simulink model "c6_formation"  (R2021b)
settings: Solver=FixedStepDiscrete  StartTime=0.0  StopTime=Inf  FixedStep=sampleTime  RelTol=1e-3  EnableMultiTasking=on
PreLoadFcn:
  | %load emptyMap
  | 
  | % Lidar parameters
  | sensorOffset = [0,0];
  | scanAngles = -pi:pi/6:pi;
  | maxRange = 0.25;
InitFcn:
  | sampleTime = 0.05;
  | nMedianSize=3;
  | 
  | % Robot parameters
  | wheelRadius = 0.0335;
  | robotRadius = 0.116/2;
  | 
  | %角速度坐标
  | ks=1;
  | 
  | % Lidar parameters
  | sensorOffset = [0,0];
  | scanAngles = -pi/3:pi/36:pi/3;
  | maxRange = 0.2;
  | 
  | %车初始位置
  | init_pose_1=[1  1.3  pi/2]';
  | init_pose_2=[0.85 1  pi/2]';
  | init_pose_3=[1.15 1  pi/2]';
  | init_pose_4=[0.7  0.7 pi/2]';
  | init_pose_5=[1  0.7 pi/2]';
  | init_pose_6=[1.3 0.7  pi/2]';
  | 
  | %pp算法性能参数
  | Vd_pp=0.2;
  | Wd_pp=pi;
  | dist_pp=0.2;
  | GoalRadius=0.1;
  | numSector=180;
  | rangeDis=[0.1,maxRange];
  | thresholds=[1/360 1/36];
  | safetyDis=0.2;
  | minimumTurningRadius=0.5*robotRadius;
  | recovery_w=0.05;
undefined symbols (not defined in the file): Angular, DiscIntNeverNeededParam, Linear
libraries: robotlib x24, dspstat3 x18, robotalgslib x6
(part 1 of 4)
settings Model: Creator=The MathWorks, Inc.  LastModifiedBy=FCS
settings SolverCC: AlgebraicLoopSolver=TrustRegion
settings DataIOCC: LimitDataPoints=on  SaveFormat=Array  ReturnWorkspaceOutputs=off
settings OptimizationCC: EnhancedBackFolding=on  PassReuseOutputArgsAs=Individual arguments  ZeroExternalMemoryAtStartup=off  ZeroInternalMemoryAtStartup=off  MaxStackSize=64  OptimizeBlockOrder=speed  DifferentSizesBufferReuse=on  OptimizationCustomize=off  EfficientTunableParamExpr=on
settings DebuggingCC: SolverPrmCheckMsg=warning  ParameterTunabilityLossMsg=error  SFUnexpectedBacktrackingDiag=warning  SFNoUnconditionalDefaultTransitionDiag=warning  SFExecutionAtInitializationDiag=none  SFMachineParentedDataDiag=warning  ArithmeticOperatorsInVariantConditions=warning
settings HardwareCC: ProdBitPerPointer=32  ProdBitPerSizeT=32  ProdBitPerPtrDiffT=32  ProdLargestAtomicFloat=None  ProdIntDivRoundTo=Undefined  ProdEndianess=Unspecified  ProdWordSize=32  ProdHWDeviceType=Generic->Unspecified (assume 32-bit Generic)  TargetHWDeviceType=Generic->Unspecified (assume 32-bit Generic)
settings ModelReferenceCC: PropagateSignalLabelsOutOfModel=off
settings SFSimCC: SimUseLocalCustomCode=off  CustomCodeUndefinedFunction=UseInterfaceOnly  SimTargetLang=C++
settings RTWCC: Description=Embedded Coder  SystemTargetFile=ert.tlc  HardwareBoard=Robot Operating System (ROS)  TLCOptions="-aInlineSetEventsForThisBaseRateFcn=TLC_FALSE -aSuppressMultiTaskScheduler=TLC_FALSE  -aRateBasedStepFcn=0"  TemplateMakefile=ert_default_tmf  RTWUseLocalCustomCode=off  Toolchain=Catkin  TargetLang=C++
settings CodeAppCC: ForceParamTrailComments=on  IgnoreCustomStorageClasses=off  OperatorAnnotations=on  SimulinkDataObjDesc=on  SFDataObjDesc=on  InsertBlockDesc=on
settings ERTTargetCC: SupportVariableSizeSignals=on
settings ConfigComp: CovMetricSettings=dw  CovSaveCumulativeToWorkspaceVar=on  CovSaveSingleToWorkspaceVar=on  CovExternalEMLEnable=off  CovSFcnEnable=off

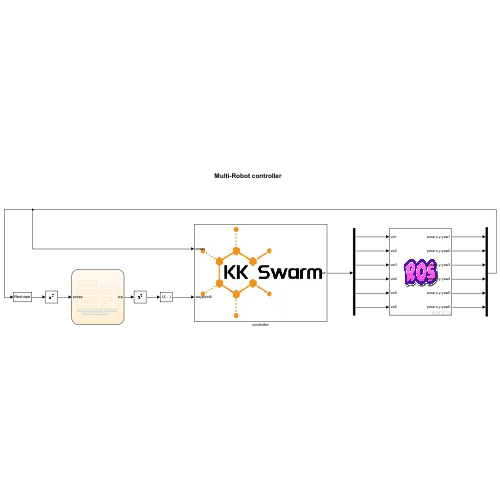
[thumbnail: Simulink's stored preview of the top-level diagram]
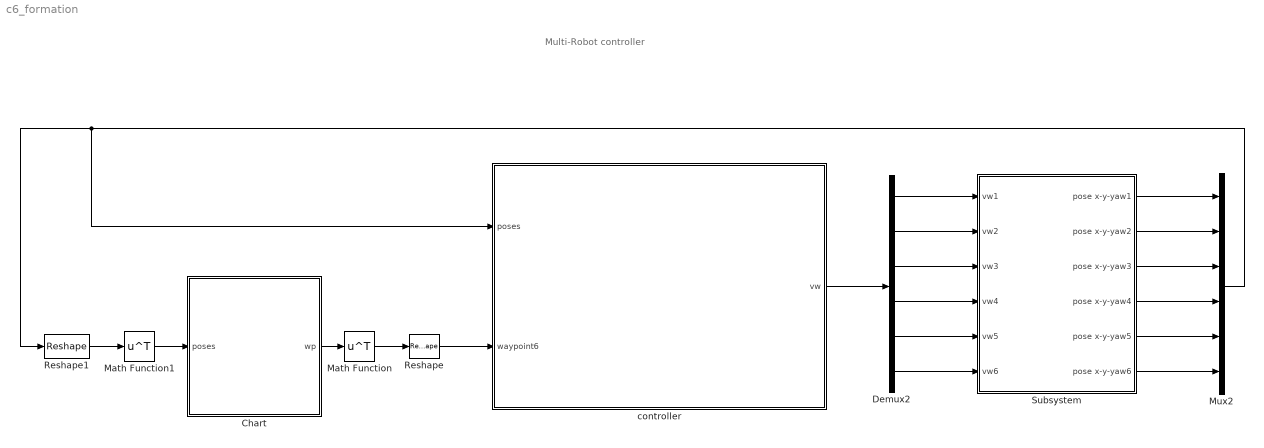
== system c6_formation ==
  note: Multi-Robot controller
  Chart : Stateflow chart  TreatAsAtomicUnit=on
  Demux2 : Demux  Outputs=6
  Math Function : Math  Operator=transpose  SaturateOnIntegerOverflow=on
  Math Function1 : Math  Operator=transpose  SaturateOnIntegerOverflow=on
  Mux2 : Mux  Inputs=6
  Reshape : Reshape
  Reshape1 : Reshape  OutputDimensionality=Customize  OutputDimensions=[3,6]
  Subsystem : Subsystem
      mask Display: image('$imagefile'); % 使用工具条上的 "编辑图像" 进行更改。
  controller : Subsystem
      mask Display: image('$imagefile'); % 使用工具条上的 "编辑图像" 进行更改。
  wires:
  Subsystem/3(pose x-y-yaw3) -> Mux2/3
  Demux2/3 -> Subsystem/3(vw3)
  Math Function/1 -> Reshape/1
  Reshape/1 -> controller/2(waypoint6)
  Subsystem/4(pose x-y-yaw4) -> Mux2/4
  Reshape1/1 -> Math Function1/1
  Mux2/1 -> Reshape1/1, controller/1(poses)
  controller/1(vw) -> Demux2/1
  Demux2/1 -> Subsystem/1(vw1)
  Demux2/2 -> Subsystem/2(vw2)
  Demux2/5 -> Subsystem/5(vw5)
  Subsystem/6(pose x-y-yaw6) -> Mux2/6
  Subsystem/2(pose x-y-yaw2) -> Mux2/2
  Demux2/4 -> Subsystem/4(vw4)
  Subsystem/1(pose x-y-yaw1) -> Mux2/1
  Demux2/6 -> Subsystem/6(vw6)
  Chart/1(wp) -> Math Function/1
  Math Function1/1 -> Chart/1(poses)
  Subsystem/5(pose x-y-yaw5) -> Mux2/5

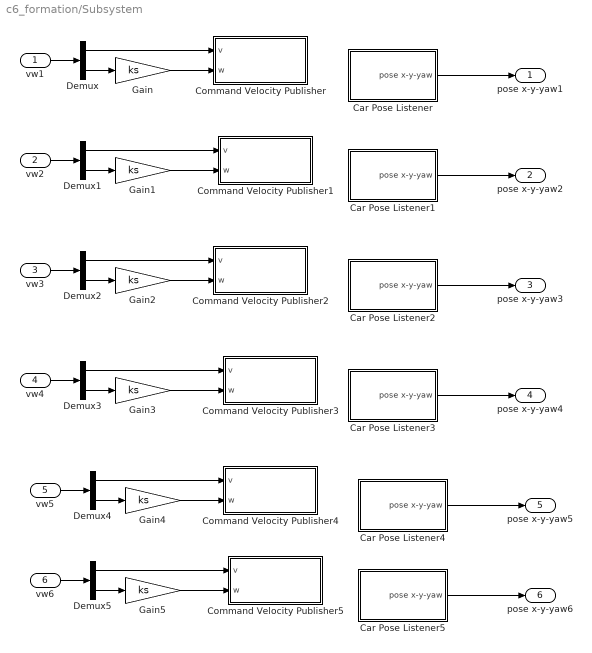
== system c6_formation/Subsystem ==
  vw1 : Inport
  vw2 : Inport  Port=2
  vw3 : Inport  Port=3
  vw4 : Inport  Port=4
  vw5 : Inport  Port=5
  vw6 : Inport  Port=6
  Car Pose Listener : Subsystem
  Car Pose Listener1 : Subsystem
  Car Pose Listener2 : Subsystem
  Car Pose Listener3 : Subsystem
  Car Pose Listener4 : Subsystem
  Car Pose Listener5 : Subsystem
  Command Velocity Publisher : Subsystem
  Command Velocity Publisher1 : Subsystem
  Command Velocity Publisher2 : Subsystem
  Command Velocity Publisher3 : Subsystem
  Command Velocity Publisher4 : Subsystem
  Command Velocity Publisher5 : Subsystem
  Demux{,1..5} (6 alike) : Demux  Outputs=2
  Gain{,1..5} (6 alike) : Gain  Gain=ks
  pose x-y-yaw1 : Outport
  pose x-y-yaw2 : Outport  Port=2
  pose x-y-yaw3 : Outport  Port=3
  pose x-y-yaw4 : Outport  Port=4
  pose x-y-yaw5 : Outport  Port=5
  pose x-y-yaw6 : Outport  Port=6
  wires:
  Gain/1 -> Command Velocity Publisher/2(w)
  Demux/2 -> Gain/1
  Car Pose Listener/1(pose x-y-yaw) -> pose x-y-yaw1/1
  Demux/1 -> Command Velocity Publisher/1(v)
  vw1/1 -> Demux/1
  Car Pose Listener1/1(pose x-y-yaw) -> pose x-y-yaw2/1
  Gain1/1 -> Command Velocity Publisher1/2(w)
  vw2/1 -> Demux1/1
  Demux1/2 -> Gain1/1
  Demux1/1 -> Command Velocity Publisher1/1(v)
  Car Pose Listener2/1(pose x-y-yaw) -> pose x-y-yaw3/1
  Gain2/1 -> Command Velocity Publisher2/2(w)
  vw3/1 -> Demux2/1
  Demux2/2 -> Gain2/1
  Demux2/1 -> Command Velocity Publisher2/1(v)
  Car Pose Listener3/1(pose x-y-yaw) -> pose x-y-yaw4/1
  Gain3/1 -> Command Velocity Publisher3/2(w)
  vw4/1 -> Demux3/1
  Demux3/2 -> Gain3/1
  Demux3/1 -> Command Velocity Publisher3/1(v)
  Car Pose Listener4/1(pose x-y-yaw) -> pose x-y-yaw5/1
  Gain4/1 -> Command Velocity Publisher4/2(w)
  vw5/1 -> Demux4/1
  Demux4/2 -> Gain4/1
  Car Pose Listener5/1(pose x-y-yaw) -> pose x-y-yaw6/1
  Gain5/1 -> Command Velocity Publisher5/2(w)
  vw6/1 -> Demux5/1
  Demux5/2 -> Gain5/1
  Demux5/1 -> Command Velocity Publisher5/1(v)
  Demux4/1 -> Command Velocity Publisher4/1(v)

== system c6_formation/controller ==
  poses : Inport
  waypoint6 : Inport  Port=2
  Car1 : Subsystem  mask{scanAngles=scanAngles, desired_v=Vd_pp, desired_w=Wd_pp, desired_lookahead=dist_pp, GoalRadius=GoalRadius, numSector=numSector, rangeDis=rangeDis, thresholds=thresholds, vehicleRadius=robotRadius, safetyDis=safetyDis, minimumTurningRadius=minimumTurningRadius, recovery_w=recovery_w}
      mask prompts: scanAngles "雷达扫描线角度"; desired_v "pp算法期望速度"; desired_w "pp算法期望角速度"; desired_lookahead "pp算法预瞄距离"; GoalRadius "到达目标的判定阈值"; numSector "直方图条柱数"; rangeDis "避障传感器距离范围"; thresholds "直方图障碍物占用空间阈值"; vehicleRadius "车辆半径"; safetyDis "车辆周边安全距离"; minimumTurningRadius "车辆的最少转弯半径"
  Car2 : Subsystem  mask{scanAngles=scanAngles, desired_v=Vd_pp, desired_w=Wd_pp, desired_lookahead=dist_pp, GoalRadius=GoalRadius, numSector=numSector, rangeDis=rangeDis, thresholds=thresholds, vehicleRadius=robotRadius, safetyDis=safetyDis, minimumTurningRadius=minimumTurningRadius, recovery_w=recovery_w}
      mask prompts: scanAngles "雷达扫描线角度"; desired_v "pp算法期望速度"; desired_w "pp算法期望角速度"; desired_lookahead "pp算法预瞄距离"; GoalRadius "到达目标的判定阈值"; numSector "直方图条柱数"; rangeDis "避障传感器距离范围"; thresholds "直方图障碍物占用空间阈值"; vehicleRadius "车辆半径"; safetyDis "车辆周边安全距离"; minimumTurningRadius "车辆的最少转弯半径"
  Car3 : Subsystem  mask{scanAngles=scanAngles, desired_v=Vd_pp, desired_w=Wd_pp, desired_lookahead=dist_pp, GoalRadius=GoalRadius, numSector=numSector, rangeDis=rangeDis, thresholds=thresholds, vehicleRadius=robotRadius, safetyDis=safetyDis, minimumTurningRadius=minimumTurningRadius, recovery_w=recovery_w}
      mask prompts: scanAngles "雷达扫描线角度"; desired_v "pp算法期望速度"; desired_w "pp算法期望角速度"; desired_lookahead "pp算法预瞄距离"; GoalRadius "到达目标的判定阈值"; numSector "直方图条柱数"; rangeDis "避障传感器距离范围"; thresholds "直方图障碍物占用空间阈值"; vehicleRadius "车辆半径"; safetyDis "车辆周边安全距离"; minimumTurningRadius "车辆的最少转弯半径"
  Car4 : Subsystem  mask{scanAngles=scanAngles, desired_v=Vd_pp, desired_w=Wd_pp, desired_lookahead=dist_pp, GoalRadius=GoalRadius, numSector=numSector, rangeDis=rangeDis, thresholds=thresholds, vehicleRadius=robotRadius, safetyDis=safetyDis, minimumTurningRadius=minimumTurningRadius, recovery_w=recovery_w}
      mask prompts: scanAngles "雷达扫描线角度"; desired_v "pp算法期望速度"; desired_w "pp算法期望角速度"; desired_lookahead "pp算法预瞄距离"; GoalRadius "到达目标的判定阈值"; numSector "直方图条柱数"; rangeDis "避障传感器距离范围"; thresholds "直方图障碍物占用空间阈值"; vehicleRadius "车辆半径"; safetyDis "车辆周边安全距离"; minimumTurningRadius "车辆的最少转弯半径"
  Car5 : Subsystem  mask{scanAngles=scanAngles, desired_v=Vd_pp, desired_w=Wd_pp, desired_lookahead=dist_pp, GoalRadius=GoalRadius, numSector=numSector, rangeDis=rangeDis, thresholds=thresholds, vehicleRadius=robotRadius, safetyDis=safetyDis, minimumTurningRadius=minimumTurningRadius, recovery_w=recovery_w}
      mask prompts: scanAngles "雷达扫描线角度"; desired_v "pp算法期望速度"; desired_w "pp算法期望角速度"; desired_lookahead "pp算法预瞄距离"; GoalRadius "到达目标的判定阈值"; numSector "直方图条柱数"; rangeDis "避障传感器距离范围"; thresholds "直方图障碍物占用空间阈值"; vehicleRadius "车辆半径"; safetyDis "车辆周边安全距离"; minimumTurningRadius "车辆的最少转弯半径"
  Car6 : Subsystem  mask{scanAngles=scanAngles, desired_v=Vd_pp, desired_w=Wd_pp, desired_lookahead=dist_pp, GoalRadius=GoalRadius, numSector=numSector, rangeDis=rangeDis, thresholds=thresholds, vehicleRadius=robotRadius, safetyDis=safetyDis, minimumTurningRadius=minimumTurningRadius, recovery_w=recovery_w}
      mask prompts: scanAngles "雷达扫描线角度"; desired_v "pp算法期望速度"; desired_w "pp算法期望角速度"; desired_lookahead "pp算法预瞄距离"; GoalRadius "到达目标的判定阈值"; numSector "直方图条柱数"; rangeDis "避障传感器距离范围"; thresholds "直方图障碍物占用空间阈值"; vehicleRadius "车辆半径"; safetyDis "车辆周边安全距离"; minimumTurningRadius "车辆的最少转弯半径"
  Demux : Demux  Outputs=6
  Demux1 : Demux  Outputs=6
  Mux : Mux  Inputs=6
  controller1 : Subsystem
      mask Display: image('$imagefile'); % 使用工具条上的 "编辑图像" 进行更改。
  vw : Outport
  wires:
  waypoint6/1 -> Demux1/1
  Mux/1 -> vw/1
  Car1/1(Out1) -> Mux/1
  poses/1 -> controller1/1(poses), Demux/1
  Car2/1(Out1) -> Mux/2
  Car6/1(Out1) -> Mux/6
  Car5/1(Out1) -> Mux/5
  Car4/1(Out1) -> Mux/4
  Car3/1(Out1) -> Mux/3
  Demux/1 -> Car1/2(Pose)
  Demux/2 -> Car2/2(Pose)
  Demux/3 -> Car3/2(Pose)
  Demux/4 -> Car4/2(Pose)
  Demux/5 -> Car5/2(Pose)
  Demux/6 -> Car6/2(Pose)
  Demux1/1 -> Car1/3(WayPoints)
  Demux1/2 -> Car2/3(WayPoints)
  Demux1/3 -> Car3/3(WayPoints)
  Demux1/4 -> Car4/3(WayPoints)
  Demux1/5 -> Car5/3(WayPoints)
  Demux1/6 -> Car6/3(WayPoints)
  controller1/1(Lidar1) -> Car1/1(Ranges)
  controller1/2(Lidar2) -> Car2/1(Ranges)
  controller1/3(Lidar3) -> Car3/1(Ranges)
  controller1/4(Lidar4) -> Car4/1(Ranges)
  controller1/5(Lidar5) -> Car5/1(Ranges)
  controller1/6(Lidar6) -> Car6/1(Ranges)

== system c6_formation/Subsystem/Car Pose Listener ==
  Subscribe : robotlib/Subscribe  topicSource=Specify your own  topic=/robot_1/pose  messageType=nav_msgs/Odometry  SampleTime=-1  legacyBusStruct=off  messageQueueLength=51
  Subscribe1 : robotlib/Subscribe  topicSource=Specify your own  topic=/robot_1/odometry  messageType=geometry_msgs/Twist  SampleTime=-1  legacyBusStruct=off  messageQueueLength=51
  Subsystem : Subsystem
  pose x-y-yaw : Outport
  wires:
  Subscribe/1 -> Subsystem/1(poseNew)  "IsNew"
  Subscribe/2 -> Subsystem/2(poseMsg)
  Subscribe1/1 -> Subsystem/3(VW_New)  "IsNew"
  Subscribe1/2 -> Subsystem/4(VW_Msg)
  Subsystem/1(pose) -> pose x-y-yaw/1

== system c6_formation/Subsystem/Car Pose Listener1 ==
  Subscribe : robotlib/Subscribe  topicSource=Specify your own  topic=/robot_2/pose  messageType=nav_msgs/Odometry  SampleTime=-1  legacyBusStruct=off  messageQueueLength=51
  Subscribe1 : robotlib/Subscribe  topicSource=Specify your own  topic=/robot_2/odometry  messageType=geometry_msgs/Twist  SampleTime=-1  legacyBusStruct=off  messageQueueLength=51
  Subsystem : Subsystem
  pose x-y-yaw : Outport
  wires:
  Subscribe/1 -> Subsystem/1(poseNew)  "IsNew"
  Subscribe/2 -> Subsystem/2(poseMsg)
  Subscribe1/2 -> Subsystem/4(VW_Msg)
  Subscribe1/1 -> Subsystem/3(VW_New)  "IsNew"
  Subsystem/1(pose) -> pose x-y-yaw/1

== system c6_formation/Subsystem/Car Pose Listener2 ==
  Subscribe : robotlib/Subscribe  topicSource=Specify your own  topic=/robot_3/pose  messageType=nav_msgs/Odometry  SampleTime=-1  legacyBusStruct=off  messageQueueLength=51
  Subscribe1 : robotlib/Subscribe  topicSource=Specify your own  topic=/robot_3/odometry  messageType=geometry_msgs/Twist  SampleTime=-1  legacyBusStruct=off  messageQueueLength=51
  Subsystem : Subsystem
  pose x-y-yaw : Outport
  wires:
  Subscribe/1 -> Subsystem/1(poseNew)  "IsNew"
  Subscribe/2 -> Subsystem/2(poseMsg)
  Subscribe1/1 -> Subsystem/3(VW_New)  "IsNew"
  Subscribe1/2 -> Subsystem/4(VW_Msg)
  Subsystem/1(pose) -> pose x-y-yaw/1

== system c6_formation/Subsystem/Car Pose Listener3 ==
  Subscribe : robotlib/Subscribe  topicSource=Specify your own  topic=/robot_4/pose  messageType=nav_msgs/Odometry  SampleTime=-1  legacyBusStruct=off  messageQueueLength=51
  Subscribe1 : robotlib/Subscribe  topicSource=Specify your own  topic=/robot_4/odometry  messageType=geometry_msgs/Twist  SampleTime=-1  legacyBusStruct=off  messageQueueLength=51
  Subsystem : Subsystem
  pose x-y-yaw : Outport
  wires:
  Subscribe/1 -> Subsystem/1(poseNew)  "IsNew"
  Subscribe/2 -> Subsystem/2(poseMsg)
  Subscribe1/1 -> Subsystem/3(VW_New)  "IsNew"
  Subscribe1/2 -> Subsystem/4(VW_Msg)
  Subsystem/1(pose) -> pose x-y-yaw/1

== system c6_formation/Subsystem/Car Pose Listener4 ==
  Subscribe : robotlib/Subscribe  topicSource=Specify your own  topic=/robot_5/pose  messageType=nav_msgs/Odometry  SampleTime=-1  legacyBusStruct=off  messageQueueLength=51
  Subscribe1 : robotlib/Subscribe  topicSource=Specify your own  topic=/robot_5/odometry  messageType=geometry_msgs/Twist  SampleTime=-1  legacyBusStruct=off  messageQueueLength=51
  Subsystem : Subsystem
  pose x-y-yaw : Outport
  wires:
  Subscribe/1 -> Subsystem/1(poseNew)  "IsNew"
  Subscribe/2 -> Subsystem/2(poseMsg)
  Subscribe1/1 -> Subsystem/3(VW_New)  "IsNew"
  Subscribe1/2 -> Subsystem/4(VW_Msg)
  Subsystem/1(pose) -> pose x-y-yaw/1

== system c6_formation/Subsystem/Car Pose Listener5 ==
  Subscribe : robotlib/Subscribe  topicSource=Specify your own  topic=/robot_6/pose  messageType=nav_msgs/Odometry  SampleTime=-1  legacyBusStruct=off  messageQueueLength=51
  Subscribe1 : robotlib/Subscribe  topicSource=Specify your own  topic=/robot_6/odometry  messageType=geometry_msgs/Twist  SampleTime=-1  legacyBusStruct=off  messageQueueLength=51
  Subsystem : Subsystem
  pose x-y-yaw : Outport
  wires:
  Subscribe/1 -> Subsystem/1(poseNew)  "IsNew"
  Subscribe/2 -> Subsystem/2(poseMsg)
  Subscribe1/1 -> Subsystem/3(VW_New)  "IsNew"
  Subscribe1/2 -> Subsystem/4(VW_Msg)
  Subsystem/1(pose) -> pose x-y-yaw/1

== system c6_formation/Subsystem/Command Velocity Publisher ==
  v : Inport
  w : Inport  Port=2
  Blank Message : robotlib/Blank Message  messageClass=Message  entityType=geometry_msgs/Twist  messageType=geometry_msgs/Twist  SampleTime=inf  legacyBusStruct=off
  Bus Assignment1 : BusAssignment  DialogController=Simulink.DDGSource_BusAssignment  AssignedSignals=Linear.X,Angular.Z
  Publish2 : robotlib/Publish  topicSource=Specify your own  topic=/robot_1/cmd_vel  messageType=geometry_msgs/Twist  legacyBusStruct=off  messageQueueLength=105
  wires:
  Bus Assignment1/1 -> Publish2/1
  Blank Message/1 -> Bus Assignment1/1
  v/1 -> Bus Assignment1/2
  w/1 -> Bus Assignment1/3

== system c6_formation/Subsystem/Command Velocity Publisher1 ==
  v : Inport
  w : Inport  Port=2
  Blank Message : robotlib/Blank Message  messageClass=Message  entityType=geometry_msgs/Twist  messageType=geometry_msgs/Twist  SampleTime=inf  legacyBusStruct=off
  Bus Assignment1 : BusAssignment  DialogController=Simulink.DDGSource_BusAssignment  AssignedSignals=Linear.X,Angular.Z
  Publish2 : robotlib/Publish  topicSource=Specify your own  topic=/robot_2/cmd_vel  messageType=geometry_msgs/Twist  legacyBusStruct=off  messageQueueLength=105
  wires:
  Bus Assignment1/1 -> Publish2/1
  Blank Message/1 -> Bus Assignment1/1
  v/1 -> Bus Assignment1/2
  w/1 -> Bus Assignment1/3

== system c6_formation/Subsystem/Command Velocity Publisher2 ==
  v : Inport
  w : Inport  Port=2
  Blank Message : robotlib/Blank Message  messageClass=Message  entityType=geometry_msgs/Twist  messageType=geometry_msgs/Twist  SampleTime=inf  legacyBusStruct=off
  Bus Assignment1 : BusAssignment  DialogController=Simulink.DDGSource_BusAssignment  AssignedSignals=Linear.X,Angular.Z
  Publish2 : robotlib/Publish  topicSource=Specify your own  topic=/robot_3/cmd_vel  messageType=geometry_msgs/Twist  legacyBusStruct=off  messageQueueLength=105
  wires:
  Bus Assignment1/1 -> Publish2/1
  Blank Message/1 -> Bus Assignment1/1
  v/1 -> Bus Assignment1/2
  w/1 -> Bus Assignment1/3

== system c6_formation/Subsystem/Command Velocity Publisher3 ==
  v : Inport
  w : Inport  Port=2
  Blank Message : robotlib/Blank Message  messageClass=Message  entityType=geometry_msgs/Twist  messageType=geometry_msgs/Twist  SampleTime=inf  legacyBusStruct=off
  Bus Assignment1 : BusAssignment  DialogController=Simulink.DDGSource_BusAssignment  AssignedSignals=Linear.X,Angular.Z
  Publish2 : robotlib/Publish  topicSource=Specify your own  topic=/robot_4/cmd_vel  messageType=geometry_msgs/Twist  legacyBusStruct=off  messageQueueLength=105
  wires:
  Bus Assignment1/1 -> Publish2/1
  Blank Message/1 -> Bus Assignment1/1
  v/1 -> Bus Assignment1/2
  w/1 -> Bus Assignment1/3

== system c6_formation/Subsystem/Command Velocity Publisher4 ==
  v : Inport
  w : Inport  Port=2
  Blank Message : robotlib/Blank Message  messageClass=Message  entityType=geometry_msgs/Twist  messageType=geometry_msgs/Twist  SampleTime=inf  legacyBusStruct=off
  Bus Assignment1 : BusAssignment  DialogController=Simulink.DDGSource_BusAssignment  AssignedSignals=Linear.X,Angular.Z
  Publish2 : robotlib/Publish  topicSource=Specify your own  topic=/robot_5/cmd_vel  messageType=geometry_msgs/Twist  legacyBusStruct=off  messageQueueLength=105
  wires:
  Bus Assignment1/1 -> Publish2/1
  Blank Message/1 -> Bus Assignment1/1
  v/1 -> Bus Assignment1/2
  w/1 -> Bus Assignment1/3

== system c6_formation/Subsystem/Command Velocity Publisher5 ==
  v : Inport
  w : Inport  Port=2
  Blank Message : robotlib/Blank Message  messageClass=Message  entityType=geometry_msgs/Twist  messageType=geometry_msgs/Twist  SampleTime=inf  legacyBusStruct=off
  Bus Assignment1 : BusAssignment  DialogController=Simulink.DDGSource_BusAssignment  AssignedSignals=Linear.X,Angular.Z
  Publish2 : robotlib/Publish  topicSource=Specify your own  topic=/robot_6/cmd_vel  messageType=geometry_msgs/Twist  legacyBusStruct=off  messageQueueLength=105
  wires:
  Bus Assignment1/1 -> Publish2/1
  Blank Message/1 -> Bus Assignment1/1
  v/1 -> Bus Assignment1/2
  w/1 -> Bus Assignment1/3

== system c6_formation/controller/Car1 ==
  Ranges : Inport
  Pose : Inport  Port=2
  WayPoints : Inport  Port=3
  Constant7 : Constant  Value=scanAngles
  Mux1 : Mux  Inputs=2
  ppCar : Subsystem
  Out1 : Outport
  wires:
  WayPoints/1 -> ppCar/4(WayPoints)
  Pose/1 -> ppCar/3(Pose)
  Ranges/1 -> ppCar/2(Ranges)
  ppCar/2(w) -> Mux1/2
  Mux1/1 -> Out1/1
  ppCar/1(v) -> Mux1/1
  Constant7/1 -> ppCar/1(Angels)

== system c6_formation/controller/Car2 ==
  Ranges : Inport
  Pose : Inport  Port=2
  WayPoints : Inport  Port=3
  Constant7 : Constant  Value=scanAngles
  Mux1 : Mux  Inputs=2
  ppCar : Subsystem
  Out1 : Outport
  wires:
  Constant7/1 -> ppCar/1(Angels)
  ppCar/1(v) -> Mux1/1
  Mux1/1 -> Out1/1
  ppCar/2(w) -> Mux1/2
  Ranges/1 -> ppCar/2(Ranges)
  Pose/1 -> ppCar/3(Pose)
  WayPoints/1 -> ppCar/4(WayPoints)

== system c6_formation/controller/Car3 ==
  Ranges : Inport
  Pose : Inport  Port=2
  WayPoints : Inport  Port=3
  Constant7 : Constant  Value=scanAngles
  Mux1 : Mux  Inputs=2
  ppCar : Subsystem
  Out1 : Outport
  wires:
  WayPoints/1 -> ppCar/4(WayPoints)
  Pose/1 -> ppCar/3(Pose)
  Ranges/1 -> ppCar/2(Ranges)
  ppCar/2(w) -> Mux1/2
  Mux1/1 -> Out1/1
  ppCar/1(v) -> Mux1/1
  Constant7/1 -> ppCar/1(Angels)

== system c6_formation/controller/Car4 ==
  Ranges : Inport
  Pose : Inport  Port=2
  WayPoints : Inport  Port=3
  Constant7 : Constant  Value=scanAngles
  Mux1 : Mux  Inputs=2
  ppCar : Subsystem
  Out1 : Outport
  wires:
  Constant7/1 -> ppCar/1(Angels)
  ppCar/1(v) -> Mux1/1
  Mux1/1 -> Out1/1
  ppCar/2(w) -> Mux1/2
  Ranges/1 -> ppCar/2(Ranges)
  Pose/1 -> ppCar/3(Pose)
  WayPoints/1 -> ppCar/4(WayPoints)

== system c6_formation/controller/Car5 ==
  Ranges : Inport
  Pose : Inport  Port=2
  WayPoints : Inport  Port=3
  Constant7 : Constant  Value=scanAngles
  Mux1 : Mux  Inputs=2
  ppCar : Subsystem
  Out1 : Outport
  wires:
  WayPoints/1 -> ppCar/4(WayPoints)
  Pose/1 -> ppCar/3(Pose)
  Ranges/1 -> ppCar/2(Ranges)
  ppCar/2(w) -> Mux1/2
  Mux1/1 -> Out1/1
  ppCar/1(v) -> Mux1/1
  Constant7/1 -> ppCar/1(Angels)

== system c6_formation/controller/Car6 ==
  Ranges : Inport
  Pose : Inport  Port=2
  WayPoints : Inport  Port=3
  Constant7 : Constant  Value=scanAngles
  Mux1 : Mux  Inputs=2
  ppCar : Subsystem
  Out1 : Outport
  wires:
  Constant7/1 -> ppCar/1(Angels)
  ppCar/1(v) -> Mux1/1
  Mux1/1 -> Out1/1
  ppCar/2(w) -> Mux1/2
  Ranges/1 -> ppCar/2(Ranges)
  Pose/1 -> ppCar/3(Pose)
  WayPoints/1 -> ppCar/4(WayPoints)

== system c6_formation/controller/controller1 ==
  poses : Inport
  Constant : Constant
  Constant1 : Constant  Value=2
  Constant2 : Constant  Value=3
  Constant3 : Constant  Value=4
  Constant4 : Constant  Value=5
  Constant5 : Constant  Value=6
  MATLAB Function1 : MATLAB Function  TreatAsAtomicUnit=on
  MATLAB Function10 : MATLAB Function  TreatAsAtomicUnit=on
  MATLAB Function2 : MATLAB Function  TreatAsAtomicUnit=on
  MATLAB Function3 : MATLAB Function  TreatAsAtomicUnit=on
  MATLAB Function4 : MATLAB Function  TreatAsAtomicUnit=on
  MATLAB Function5 : MATLAB Function  TreatAsAtomicUnit=on
  Reshape1 : Reshape  OutputDimensionality=Customize  OutputDimensions=[3,6]
  Lidar1 : Outport
  Lidar2 : Outport  Port=2
  Lidar3 : Outport  Port=3
  Lidar4 : Outport  Port=4
  Lidar5 : Outport  Port=5
  Lidar6 : Outport  Port=6
  wires:
  poses/1 -> Reshape1/1
  MATLAB Function10/1(ranges) -> Lidar1/1
  Constant/1 -> MATLAB Function10/2(idx)
  Constant1/1 -> MATLAB Function5/2(idx)
  Constant2/1 -> MATLAB Function1/2(idx)
  Reshape1/1 -> MATLAB Function5/1(poses), MATLAB Function1/1(poses), MATLAB Function2/1(poses), MATLAB Function3/1(poses), MATLAB Function4/1(poses), MATLAB Function10/1(poses)
  MATLAB Function5/1(ranges) -> Lidar2/1
  MATLAB Function1/1(ranges) -> Lidar3/1
  MATLAB Function2/1(ranges) -> Lidar4/1
  MATLAB Function3/1(ranges) -> Lidar5/1
  MATLAB Function4/1(ranges) -> Lidar6/1
  Constant3/1 -> MATLAB Function2/2(idx)
  Constant5/1 -> MATLAB Function4/2(idx)
  Constant4/1 -> MATLAB Function3/2(idx)

== system c6_formation/Subsystem/Car Pose Listener/Subsystem ==
  poseNew : Inport
  poseMsg : Inport  Port=2
  VW_New : Inport  Port=3
  VW_Msg : Inport  Port=4
  DiffSteer Kinematics : Subsystem
      settings: PortSchema="{\"entries\":[{\"content\":{\"sides\":[{\"content\":{\"connectorIds\":[\"In1\",\"In2\"]},\"type\":\"ConnectorPlacement.EquallySpacedRectSide\",\"uuid\":\"0032ed68-1de4-4b1c-b237-9372fedc8a7a\"},{\"content\":{\"connectorIds\":[\"Out1\",\"Out2\",\"Out3\"],\"side\":\"RIGHT\"},\"type\":\"ConnectorPlacement.EquallySpacedRectSide\",\"uuid\":\"d0c861bd-7497-47fe-b183-36da470ee2c6\"},{\"content\":{\"connectorIds\":[\"In3\",\"In4\"],\"side\":\"TOP\"},\"type\":\"ConnectorPlacement.EquallySpacedRectSide\",\"uuid\":\"5b685229-150b-4cb5-b33d-c61d28c4627e\"}]},\"type\":\"ConnectorPlacement.EquallySpacedConnector\",\"uuid\":\"4513c50b-5820-40cb-bb28-cc7c1b1322fe\"}],\"packageUris\":[\"http://schema.mathworks.com/mf0/Connector/R2020b\"],\"version\":\"1.0\"}"
  Median Filter : dspstat3/Median Filter  WindowLength=nMedianSize  SimulateUsing=Interpreted execution
      settings: SourceProductBaseCode=DS
  Median Filter1 : dspstat3/Median Filter  WindowLength=nMedianSize  SimulateUsing=Interpreted execution
      settings: SourceProductBaseCode=DS
  Median Filter2 : dspstat3/Median Filter  WindowLength=nMedianSize  SimulateUsing=Interpreted execution
      settings: SourceProductBaseCode=DS
  Mux7 : Mux  Inputs=3
  Sum : Sum  Inputs=++|
  Sum1 : Sum  Inputs=++|
  sensor2vCar : MATLAB Function  TreatAsAtomicUnit=on
  sensor2vCar4 : MATLAB Function  TreatAsAtomicUnit=on
  pose : Outport
  wires:
  Median Filter2/1 -> Mux7/3
  Median Filter1/1 -> Mux7/2
  Median Filter/1 -> Mux7/1
  sensor2vCar/4(flag) -> DiffSteer Kinematics/3(reset)
  DiffSteer Kinematics/2(y) -> Sum1/2
  sensor2vCar/3(yaw_init) -> DiffSteer Kinematics/4(yaw0)
  sensor2vCar/2(y_init) -> Sum1/1
  sensor2vCar/1(x_init) -> Sum/1
  DiffSteer Kinematics/1(x) -> Sum/2
  VW_New/1 -> sensor2vCar4/1(VW_New)
  Mux7/1 -> pose/1
  Sum/1 -> Median Filter/1
  DiffSteer Kinematics/3(psi) -> Median Filter2/1
  sensor2vCar4/1(V) -> DiffSteer Kinematics/1(u)
  Sum1/1 -> Median Filter1/1
  sensor2vCar4/2(W) -> DiffSteer Kinematics/2(w)
  poseNew/1 -> sensor2vCar/1(poseNew)
  poseMsg/1 -> sensor2vCar/2(poseMsg)
  VW_Msg/1 -> sensor2vCar4/2(VW_Msg)

== system c6_formation/Subsystem/Car Pose Listener1/Subsystem ==
  poseNew : Inport
  poseMsg : Inport  Port=2
  VW_New : Inport  Port=3
  VW_Msg : Inport  Port=4
  DiffSteer Kinematics : Subsystem
      settings: PortSchema="{\"entries\":[{\"content\":{\"sides\":[{\"content\":{\"connectorIds\":[\"In1\",\"In2\"]},\"type\":\"ConnectorPlacement.EquallySpacedRectSide\",\"uuid\":\"0032ed68-1de4-4b1c-b237-9372fedc8a7a\"},{\"content\":{\"connectorIds\":[\"Out1\",\"Out2\",\"Out3\"],\"side\":\"RIGHT\"},\"type\":\"ConnectorPlacement.EquallySpacedRectSide\",\"uuid\":\"d0c861bd-7497-47fe-b183-36da470ee2c6\"},{\"content\":{\"connectorIds\":[\"In3\",\"In4\"],\"side\":\"TOP\"},\"type\":\"ConnectorPlacement.EquallySpacedRectSide\",\"uuid\":\"5b685229-150b-4cb5-b33d-c61d28c4627e\"}]},\"type\":\"ConnectorPlacement.EquallySpacedConnector\",\"uuid\":\"4513c50b-5820-40cb-bb28-cc7c1b1322fe\"}],\"packageUris\":[\"http://schema.mathworks.com/mf0/Connector/R2020b\"],\"version\":\"1.0\"}"
  Median Filter : dspstat3/Median Filter  WindowLength=nMedianSize  SimulateUsing=Interpreted execution
      settings: SourceProductBaseCode=DS
  Median Filter1 : dspstat3/Median Filter  WindowLength=nMedianSize  SimulateUsing=Interpreted execution
      settings: SourceProductBaseCode=DS
  Median Filter2 : dspstat3/Median Filter  WindowLength=nMedianSize  SimulateUsing=Interpreted execution
      settings: SourceProductBaseCode=DS
  Mux7 : Mux  Inputs=3
  Sum : Sum  Inputs=++|
  Sum1 : Sum  Inputs=++|
  sensor2vCar : MATLAB Function  TreatAsAtomicUnit=on
  sensor2vCar4 : MATLAB Function  TreatAsAtomicUnit=on
  pose : Outport
  wires:
  Median Filter2/1 -> Mux7/3
  Median Filter1/1 -> Mux7/2
  Median Filter/1 -> Mux7/1
  sensor2vCar/4(flag) -> DiffSteer Kinematics/3(reset)
  DiffSteer Kinematics/2(y) -> Sum1/2
  sensor2vCar/3(yaw_init) -> DiffSteer Kinematics/4(yaw0)
  sensor2vCar/2(y_init) -> Sum1/1
  sensor2vCar/1(x_init) -> Sum/1
  DiffSteer Kinematics/1(x) -> Sum/2
  VW_New/1 -> sensor2vCar4/1(VW_New)
  Mux7/1 -> pose/1
  Sum/1 -> Median Filter/1
  DiffSteer Kinematics/3(psi) -> Median Filter2/1
  sensor2vCar4/1(V) -> DiffSteer Kinematics/1(u)
  Sum1/1 -> Median Filter1/1
  sensor2vCar4/2(W) -> DiffSteer Kinematics/2(w)
  poseNew/1 -> sensor2vCar/1(poseNew)
  poseMsg/1 -> sensor2vCar/2(poseMsg)
  VW_Msg/1 -> sensor2vCar4/2(VW_Msg)

== system c6_formation/Subsystem/Car Pose Listener2/Subsystem ==
  poseNew : Inport
  poseMsg : Inport  Port=2
  VW_New : Inport  Port=3
  VW_Msg : Inport  Port=4
  DiffSteer Kinematics : Subsystem
      settings: PortSchema="{\"entries\":[{\"content\":{\"sides\":[{\"content\":{\"connectorIds\":[\"In1\",\"In2\"]},\"type\":\"ConnectorPlacement.EquallySpacedRectSide\",\"uuid\":\"0032ed68-1de4-4b1c-b237-9372fedc8a7a\"},{\"content\":{\"connectorIds\":[\"Out1\",\"Out2\",\"Out3\"],\"side\":\"RIGHT\"},\"type\":\"ConnectorPlacement.EquallySpacedRectSide\",\"uuid\":\"d0c861bd-7497-47fe-b183-36da470ee2c6\"},{\"content\":{\"connectorIds\":[\"In3\",\"In4\"],\"side\":\"TOP\"},\"type\":\"ConnectorPlacement.EquallySpacedRectSide\",\"uuid\":\"5b685229-150b-4cb5-b33d-c61d28c4627e\"}]},\"type\":\"ConnectorPlacement.EquallySpacedConnector\",\"uuid\":\"4513c50b-5820-40cb-bb28-cc7c1b1322fe\"}],\"packageUris\":[\"http://schema.mathworks.com/mf0/Connector/R2020b\"],\"version\":\"1.0\"}"
  Median Filter : dspstat3/Median Filter  WindowLength=nMedianSize  SimulateUsing=Interpreted execution
      settings: SourceProductBaseCode=DS
  Median Filter1 : dspstat3/Median Filter  WindowLength=nMedianSize  SimulateUsing=Interpreted execution
      settings: SourceProductBaseCode=DS
  Median Filter2 : dspstat3/Median Filter  WindowLength=nMedianSize  SimulateUsing=Interpreted execution
      settings: SourceProductBaseCode=DS
  Mux7 : Mux  Inputs=3
  Sum : Sum  Inputs=++|
  Sum1 : Sum  Inputs=++|
  sensor2vCar : MATLAB Function  TreatAsAtomicUnit=on
  sensor2vCar4 : MATLAB Function  TreatAsAtomicUnit=on
  pose : Outport
  wires:
  Median Filter2/1 -> Mux7/3
  Median Filter1/1 -> Mux7/2
  Median Filter/1 -> Mux7/1
  sensor2vCar/4(flag) -> DiffSteer Kinematics/3(reset)
  DiffSteer Kinematics/2(y) -> Sum1/2
  sensor2vCar/3(yaw_init) -> DiffSteer Kinematics/4(yaw0)
  sensor2vCar/2(y_init) -> Sum1/1
  sensor2vCar/1(x_init) -> Sum/1
  DiffSteer Kinematics/1(x) -> Sum/2
  VW_New/1 -> sensor2vCar4/1(VW_New)
  Mux7/1 -> pose/1
  Sum/1 -> Median Filter/1
  DiffSteer Kinematics/3(psi) -> Median Filter2/1
  sensor2vCar4/1(V) -> DiffSteer Kinematics/1(u)
  Sum1/1 -> Median Filter1/1
  sensor2vCar4/2(W) -> DiffSteer Kinematics/2(w)
  poseNew/1 -> sensor2vCar/1(poseNew)
  poseMsg/1 -> sensor2vCar/2(poseMsg)
  VW_Msg/1 -> sensor2vCar4/2(VW_Msg)

== system c6_formation/Subsystem/Car Pose Listener3/Subsystem ==
  poseNew : Inport
  poseMsg : Inport  Port=2
  VW_New : Inport  Port=3
  VW_Msg : Inport  Port=4
  DiffSteer Kinematics : Subsystem
      settings: PortSchema="{\"entries\":[{\"content\":{\"sides\":[{\"content\":{\"connectorIds\":[\"In1\",\"In2\"]},\"type\":\"ConnectorPlacement.EquallySpacedRectSide\",\"uuid\":\"0032ed68-1de4-4b1c-b237-9372fedc8a7a\"},{\"content\":{\"connectorIds\":[\"Out1\",\"Out2\",\"Out3\"],\"side\":\"RIGHT\"},\"type\":\"ConnectorPlacement.EquallySpacedRectSide\",\"uuid\":\"d0c861bd-7497-47fe-b183-36da470ee2c6\"},{\"content\":{\"connectorIds\":[\"In3\",\"In4\"],\"side\":\"TOP\"},\"type\":\"ConnectorPlacement.EquallySpacedRectSide\",\"uuid\":\"5b685229-150b-4cb5-b33d-c61d28c4627e\"}]},\"type\":\"ConnectorPlacement.EquallySpacedConnector\",\"uuid\":\"4513c50b-5820-40cb-bb28-cc7c1b1322fe\"}],\"packageUris\":[\"http://schema.mathworks.com/mf0/Connector/R2020b\"],\"version\":\"1.0\"}"
  Median Filter : dspstat3/Median Filter  WindowLength=nMedianSize  SimulateUsing=Interpreted execution
      settings: SourceProductBaseCode=DS
  Median Filter1 : dspstat3/Median Filter  WindowLength=nMedianSize  SimulateUsing=Interpreted execution
      settings: SourceProductBaseCode=DS
  Median Filter2 : dspstat3/Median Filter  WindowLength=nMedianSize  SimulateUsing=Interpreted execution
      settings: SourceProductBaseCode=DS
  Mux7 : Mux  Inputs=3
  Sum : Sum  Inputs=++|
  Sum1 : Sum  Inputs=++|
  sensor2vCar : MATLAB Function  TreatAsAtomicUnit=on
  sensor2vCar4 : MATLAB Function  TreatAsAtomicUnit=on
  pose : Outport
  wires:
  Median Filter2/1 -> Mux7/3
  Median Filter1/1 -> Mux7/2
  Median Filter/1 -> Mux7/1
  sensor2vCar/4(flag) -> DiffSteer Kinematics/3(reset)
  DiffSteer Kinematics/2(y) -> Sum1/2
  sensor2vCar/3(yaw_init) -> DiffSteer Kinematics/4(yaw0)
  sensor2vCar/2(y_init) -> Sum1/1
  sensor2vCar/1(x_init) -> Sum/1
  DiffSteer Kinematics/1(x) -> Sum/2
  VW_New/1 -> sensor2vCar4/1(VW_New)
  Mux7/1 -> pose/1
  Sum/1 -> Median Filter/1
  DiffSteer Kinematics/3(psi) -> Median Filter2/1
  sensor2vCar4/1(V) -> DiffSteer Kinematics/1(u)
  Sum1/1 -> Median Filter1/1
  sensor2vCar4/2(W) -> DiffSteer Kinematics/2(w)
  poseNew/1 -> sensor2vCar/1(poseNew)
  poseMsg/1 -> sensor2vCar/2(poseMsg)
  VW_Msg/1 -> sensor2vCar4/2(VW_Msg)

== system c6_formation/Subsystem/Car Pose Listener4/Subsystem ==
  poseNew : Inport
  poseMsg : Inport  Port=2
  VW_New : Inport  Port=3
  VW_Msg : Inport  Port=4
  DiffSteer Kinematics : Subsystem
      settings: PortSchema="{\"entries\":[{\"content\":{\"sides\":[{\"content\":{\"connectorIds\":[\"In1\",\"In2\"]},\"type\":\"ConnectorPlacement.EquallySpacedRectSide\",\"uuid\":\"0032ed68-1de4-4b1c-b237-9372fedc8a7a\"},{\"content\":{\"connectorIds\":[\"Out1\",\"Out2\",\"Out3\"],\"side\":\"RIGHT\"},\"type\":\"ConnectorPlacement.EquallySpacedRectSide\",\"uuid\":\"d0c861bd-7497-47fe-b183-36da470ee2c6\"},{\"content\":{\"connectorIds\":[\"In3\",\"In4\"],\"side\":\"TOP\"},\"type\":\"ConnectorPlacement.EquallySpacedRectSide\",\"uuid\":\"5b685229-150b-4cb5-b33d-c61d28c4627e\"}]},\"type\":\"ConnectorPlacement.EquallySpacedConnector\",\"uuid\":\"4513c50b-5820-40cb-bb28-cc7c1b1322fe\"}],\"packageUris\":[\"http://schema.mathworks.com/mf0/Connector/R2020b\"],\"version\":\"1.0\"}"
  Median Filter : dspstat3/Median Filter  WindowLength=nMedianSize  SimulateUsing=Interpreted execution
      settings: SourceProductBaseCode=DS
  Median Filter1 : dspstat3/Median Filter  WindowLength=nMedianSize  SimulateUsing=Interpreted execution
      settings: SourceProductBaseCode=DS
  Median Filter2 : dspstat3/Median Filter  WindowLength=nMedianSize  SimulateUsing=Interpreted execution
      settings: SourceProductBaseCode=DS
  Mux7 : Mux  Inputs=3
  Sum : Sum  Inputs=++|
  Sum1 : Sum  Inputs=++|
  sensor2vCar : MATLAB Function  TreatAsAtomicUnit=on
  sensor2vCar4 : MATLAB Function  TreatAsAtomicUnit=on
  pose : Outport
  wires:
  Median Filter2/1 -> Mux7/3
  Median Filter1/1 -> Mux7/2
  Median Filter/1 -> Mux7/1
  sensor2vCar/4(flag) -> DiffSteer Kinematics/3(reset)
  DiffSteer Kinematics/2(y) -> Sum1/2
  sensor2vCar/3(yaw_init) -> DiffSteer Kinematics/4(yaw0)
  sensor2vCar/2(y_init) -> Sum1/1
  sensor2vCar/1(x_init) -> Sum/1
  DiffSteer Kinematics/1(x) -> Sum/2
  VW_New/1 -> sensor2vCar4/1(VW_New)
  Mux7/1 -> pose/1
  Sum/1 -> Median Filter/1
  DiffSteer Kinematics/3(psi) -> Median Filter2/1
  sensor2vCar4/1(V) -> DiffSteer Kinematics/1(u)
  Sum1/1 -> Median Filter1/1
  sensor2vCar4/2(W) -> DiffSteer Kinematics/2(w)
  poseNew/1 -> sensor2vCar/1(poseNew)
  poseMsg/1 -> sensor2vCar/2(poseMsg)
  VW_Msg/1 -> sensor2vCar4/2(VW_Msg)

== system c6_formation/Subsystem/Car Pose Listener5/Subsystem ==
  poseNew : Inport
  poseMsg : Inport  Port=2
  VW_New : Inport  Port=3
  VW_Msg : Inport  Port=4
  DiffSteer Kinematics : Subsystem
      settings: PortSchema="{\"entries\":[{\"content\":{\"sides\":[{\"content\":{\"connectorIds\":[\"In1\",\"In2\"]},\"type\":\"ConnectorPlacement.EquallySpacedRectSide\",\"uuid\":\"0032ed68-1de4-4b1c-b237-9372fedc8a7a\"},{\"content\":{\"connectorIds\":[\"Out1\",\"Out2\",\"Out3\"],\"side\":\"RIGHT\"},\"type\":\"ConnectorPlacement.EquallySpacedRectSide\",\"uuid\":\"d0c861bd-7497-47fe-b183-36da470ee2c6\"},{\"content\":{\"connectorIds\":[\"In3\",\"In4\"],\"side\":\"TOP\"},\"type\":\"ConnectorPlacement.EquallySpacedRectSide\",\"uuid\":\"5b685229-150b-4cb5-b33d-c61d28c4627e\"}]},\"type\":\"ConnectorPlacement.EquallySpacedConnector\",\"uuid\":\"4513c50b-5820-40cb-bb28-cc7c1b1322fe\"}],\"packageUris\":[\"http://schema.mathworks.com/mf0/Connector/R2020b\"],\"version\":\"1.0\"}"
  Median Filter : dspstat3/Median Filter  WindowLength=nMedianSize  SimulateUsing=Interpreted execution
      settings: SourceProductBaseCode=DS
  Median Filter1 : dspstat3/Median Filter  WindowLength=nMedianSize  SimulateUsing=Interpreted execution
      settings: SourceProductBaseCode=DS
  Median Filter2 : dspstat3/Median Filter  WindowLength=nMedianSize  SimulateUsing=Interpreted execution
      settings: SourceProductBaseCode=DS
  Mux7 : Mux  Inputs=3
  Sum : Sum  Inputs=++|
  Sum1 : Sum  Inputs=++|
  sensor2vCar : MATLAB Function  TreatAsAtomicUnit=on
  sensor2vCar4 : MATLAB Function  TreatAsAtomicUnit=on
  pose : Outport
  wires:
  Median Filter2/1 -> Mux7/3
  Median Filter1/1 -> Mux7/2
  Median Filter/1 -> Mux7/1
  sensor2vCar/4(flag) -> DiffSteer Kinematics/3(reset)
  DiffSteer Kinematics/2(y) -> Sum1/2
  sensor2vCar/3(yaw_init) -> DiffSteer Kinematics/4(yaw0)
  sensor2vCar/2(y_init) -> Sum1/1
  sensor2vCar/1(x_init) -> Sum/1
  DiffSteer Kinematics/1(x) -> Sum/2
  VW_New/1 -> sensor2vCar4/1(VW_New)
  Mux7/1 -> pose/1
  Sum/1 -> Median Filter/1
  DiffSteer Kinematics/3(psi) -> Median Filter2/1
  sensor2vCar4/1(V) -> DiffSteer Kinematics/1(u)
  Sum1/1 -> Median Filter1/1
  sensor2vCar4/2(W) -> DiffSteer Kinematics/2(w)
  poseNew/1 -> sensor2vCar/1(poseNew)
  poseMsg/1 -> sensor2vCar/2(poseMsg)
  VW_Msg/1 -> sensor2vCar4/2(VW_Msg)

== system c6_formation/controller/Car1/ppCar ==
  note: Path Following with Obstacle Avoidance in Simulink
  Angels : Inport
  Ranges : Inport  Port=2
  Pose : Inport  Port=3
  WayPoints : Inport  Port=4
  Adjust Velocities to Avoid Obstacles : Subsystem
  Compute Velocity and Heading for Path following : Subsystem
  Constant1 : Constant  Value=scanAngles
  More Info : Subsystem
      settings: OpenFcn=showdemo(bdroot(gcb))
      mask Display: disp('?')
  Outputs : Subsystem
  v : Outport
  w : Outport  Port=2
  wires:
  Outputs/2(w) -> w/1
  Outputs/1(v) -> v/1
  Adjust Velocities to Avoid Obstacles/1(dV) -> Outputs/1(dV)
  WayPoints/1 -> Compute Velocity and Heading for Path following/2(Waypoints)
  Ranges/1 -> Adjust Velocities to Avoid Obstacles/1(Ranges)
  Compute Velocity and Heading for Path following/2(V) -> Outputs/3(V), Adjust Velocities to Avoid Obstacles/4(V)
  Adjust Velocities to Avoid Obstacles/2(dW) -> Outputs/2(dW)
  Pose/1 -> Compute Velocity and Heading for Path following/1(CurrentPose)
  Compute Velocity and Heading for Path following/3(W) -> Outputs/4(W), Adjust Velocities to Avoid Obstacles/5(W)
  Compute Velocity and Heading for Path following/1(TargetDir) -> Adjust Velocities to Avoid Obstacles/3(TargetDir)
  Angels/1 -> Adjust Velocities to Avoid Obstacles/2(Angles)

== system c6_formation/controller/Car2/ppCar ==
  note: Path Following with Obstacle Avoidance in Simulink
  Angels : Inport
  Ranges : Inport  Port=2
  Pose : Inport  Port=3
  WayPoints : Inport  Port=4
  Adjust Velocities to Avoid Obstacles : Subsystem
  Compute Velocity and Heading for Path following : Subsystem
  Constant1 : Constant  Value=scanAngles
  More Info : Subsystem
      settings: OpenFcn=showdemo(bdroot(gcb))
      mask Display: disp('?')
  Outputs : Subsystem
  v : Outport
  w : Outport  Port=2
  wires:
  Angels/1 -> Adjust Velocities to Avoid Obstacles/2(Angles)
  Compute Velocity and Heading for Path following/1(TargetDir) -> Adjust Velocities to Avoid Obstacles/3(TargetDir)
  Compute Velocity and Heading for Path following/3(W) -> Adjust Velocities to Avoid Obstacles/5(W), Outputs/4(W)
  Pose/1 -> Compute Velocity and Heading for Path following/1(CurrentPose)
  Adjust Velocities to Avoid Obstacles/2(dW) -> Outputs/2(dW)
  Compute Velocity and Heading for Path following/2(V) -> Adjust Velocities to Avoid Obstacles/4(V), Outputs/3(V)
  Ranges/1 -> Adjust Velocities to Avoid Obstacles/1(Ranges)
  WayPoints/1 -> Compute Velocity and Heading for Path following/2(Waypoints)
  Adjust Velocities to Avoid Obstacles/1(dV) -> Outputs/1(dV)
  Outputs/1(v) -> v/1
  Outputs/2(w) -> w/1

== system c6_formation/controller/Car3/ppCar ==
  note: Path Following with Obstacle Avoidance in Simulink
  Angels : Inport
  Ranges : Inport  Port=2
  Pose : Inport  Port=3
  WayPoints : Inport  Port=4
  Adjust Velocities to Avoid Obstacles : Subsystem
  Compute Velocity and Heading for Path following : Subsystem
  Constant1 : Constant  Value=scanAngles
  More Info : Subsystem
      settings: OpenFcn=showdemo(bdroot(gcb))
      mask Display: disp('?')
  Outputs : Subsystem
  v : Outport
  w : Outport  Port=2
  wires:
  Outputs/2(w) -> w/1
  Outputs/1(v) -> v/1
  Adjust Velocities to Avoid Obstacles/1(dV) -> Outputs/1(dV)
  WayPoints/1 -> Compute Velocity and Heading for Path following/2(Waypoints)
  Ranges/1 -> Adjust Velocities to Avoid Obstacles/1(Ranges)
  Compute Velocity and Heading for Path following/2(V) -> Outputs/3(V), Adjust Velocities to Avoid Obstacles/4(V)
  Adjust Velocities to Avoid Obstacles/2(dW) -> Outputs/2(dW)
  Pose/1 -> Compute Velocity and Heading for Path following/1(CurrentPose)
  Compute Velocity and Heading for Path following/3(W) -> Outputs/4(W), Adjust Velocities to Avoid Obstacles/5(W)
  Compute Velocity and Heading for Path following/1(TargetDir) -> Adjust Velocities to Avoid Obstacles/3(TargetDir)
  Angels/1 -> Adjust Velocities to Avoid Obstacles/2(Angles)

== system c6_formation/controller/Car4/ppCar ==
  note: Path Following with Obstacle Avoidance in Simulink
  Angels : Inport
  Ranges : Inport  Port=2
  Pose : Inport  Port=3
  WayPoints : Inport  Port=4
  Adjust Velocities to Avoid Obstacles : Subsystem
  Compute Velocity and Heading for Path following : Subsystem
  Constant1 : Constant  Value=scanAngles
  More Info : Subsystem
      settings: OpenFcn=showdemo(bdroot(gcb))
      mask Display: disp('?')
  Outputs : Subsystem
  v : Outport
  w : Outport  Port=2
  wires:
  Angels/1 -> Adjust Velocities to Avoid Obstacles/2(Angles)
  Compute Velocity and Heading for Path following/1(TargetDir) -> Adjust Velocities to Avoid Obstacles/3(TargetDir)
  Compute Velocity and Heading for Path following/3(W) -> Adjust Velocities to Avoid Obstacles/5(W), Outputs/4(W)
  Pose/1 -> Compute Velocity and Heading for Path following/1(CurrentPose)
  Adjust Velocities to Avoid Obstacles/2(dW) -> Outputs/2(dW)
  Compute Velocity and Heading for Path following/2(V) -> Adjust Velocities to Avoid Obstacles/4(V), Outputs/3(V)
  Ranges/1 -> Adjust Velocities to Avoid Obstacles/1(Ranges)
  WayPoints/1 -> Compute Velocity and Heading for Path following/2(Waypoints)
  Adjust Velocities to Avoid Obstacles/1(dV) -> Outputs/1(dV)
  Outputs/1(v) -> v/1
  Outputs/2(w) -> w/1

== system c6_formation/controller/Car5/ppCar ==
  note: Path Following with Obstacle Avoidance in Simulink
  Angels : Inport
  Ranges : Inport  Port=2
  Pose : Inport  Port=3
  WayPoints : Inport  Port=4
  Adjust Velocities to Avoid Obstacles : Subsystem
  Compute Velocity and Heading for Path following : Subsystem
  Constant1 : Constant  Value=scanAngles
  More Info : Subsystem
      settings: OpenFcn=showdemo(bdroot(gcb))
      mask Display: disp('?')
  Outputs : Subsystem
  v : Outport
  w : Outport  Port=2
  wires:
  Outputs/2(w) -> w/1
  Outputs/1(v) -> v/1
  Adjust Velocities to Avoid Obstacles/1(dV) -> Outputs/1(dV)
  WayPoints/1 -> Compute Velocity and Heading for Path following/2(Waypoints)
  Ranges/1 -> Adjust Velocities to Avoid Obstacles/1(Ranges)
  Compute Velocity and Heading for Path following/2(V) -> Outputs/3(V), Adjust Velocities to Avoid Obstacles/4(V)
  Adjust Velocities to Avoid Obstacles/2(dW) -> Outputs/2(dW)
  Pose/1 -> Compute Velocity and Heading for Path following/1(CurrentPose)
  Compute Velocity and Heading for Path following/3(W) -> Outputs/4(W), Adjust Velocities to Avoid Obstacles/5(W)
  Compute Velocity and Heading for Path following/1(TargetDir) -> Adjust Velocities to Avoid Obstacles/3(TargetDir)
  Angels/1 -> Adjust Velocities to Avoid Obstacles/2(Angles)

== system c6_formation/controller/Car6/ppCar ==
  note: Path Following with Obstacle Avoidance in Simulink
  Angels : Inport
  Ranges : Inport  Port=2
  Pose : Inport  Port=3
  WayPoints : Inport  Port=4
  Adjust Velocities to Avoid Obstacles : Subsystem
  Compute Velocity and Heading for Path following : Subsystem
  Constant1 : Constant  Value=scanAngles
  More Info : Subsystem
      settings: OpenFcn=showdemo(bdroot(gcb))
      mask Display: disp('?')
  Outputs : Subsystem
  v : Outport
  w : Outport  Port=2
  wires:
  Angels/1 -> Adjust Velocities to Avoid Obstacles/2(Angles)
  Compute Velocity and Heading for Path following/1(TargetDir) -> Adjust Velocities to Avoid Obstacles/3(TargetDir)
  Compute Velocity and Heading for Path following/3(W) -> Adjust Velocities to Avoid Obstacles/5(W), Outputs/4(W)
  Pose/1 -> Compute Velocity and Heading for Path following/1(CurrentPose)
  Adjust Velocities to Avoid Obstacles/2(dW) -> Outputs/2(dW)
  Compute Velocity and Heading for Path following/2(V) -> Adjust Velocities to Avoid Obstacles/4(V), Outputs/3(V)
  Ranges/1 -> Adjust Velocities to Avoid Obstacles/1(Ranges)
  WayPoints/1 -> Compute Velocity and Heading for Path following/2(Waypoints)
  Adjust Velocities to Avoid Obstacles/1(dV) -> Outputs/1(dV)
  Outputs/1(v) -> v/1
  Outputs/2(w) -> w/1

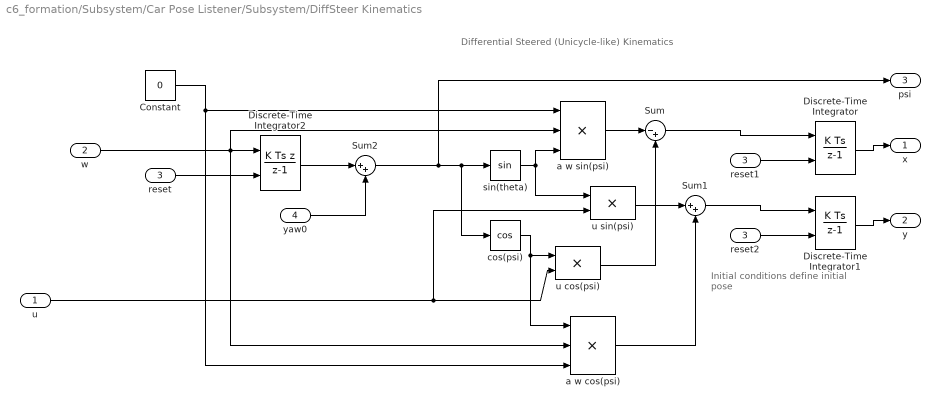
== system c6_formation/Subsystem/Car Pose Listener/Subsystem/DiffSteer Kinematics ==
  note: Initial conditions define
      | initial pose
  note: Differential Steered (Unicycle-like) Kinematics
  u : Inport
  w : Inport  Port=2
  reset : Inport  Port=3
  yaw0 : Inport  Port=4
  Constant : Constant  Value=0
  Discrete-Time Integrator : DiscreteIntegrator  ExternalReset=falling  SampleTime=-1  ICPrevOutput=DiscIntNeverNeededParam  ICPrevScaledInput=DiscIntNeverNeededParam
  Discrete-Time Integrator1 : DiscreteIntegrator  ExternalReset=falling  SampleTime=-1  ICPrevOutput=DiscIntNeverNeededParam  ICPrevScaledInput=DiscIntNeverNeededParam
  Discrete-Time Integrator2 : DiscreteIntegrator  IntegratorMethod=Integration: Backward Euler  ExternalReset=falling  SampleTime=-1  ICPrevOutput=DiscIntNeverNeededParam  ICPrevScaledInput=DiscIntNeverNeededParam
  Sum : Sum  Inputs=|-+  SaturateOnIntegerOverflow=on
  Sum1 : Sum  Inputs=|++  SaturateOnIntegerOverflow=on
  Sum2 : Sum  Inputs=|++
  a w cos(psi) : Product  Inputs=3  SaturateOnIntegerOverflow=on  OutDataTypeStr=Inherit: Same as first input
  a w sin(psi) : Product  Inputs=3  SaturateOnIntegerOverflow=on  OutDataTypeStr=Inherit: Same as first input
  cos(psi) : Trigonometry  Operator=cos
  reset1 : InportShadow  Port=3
  reset2 : InportShadow  Port=3
  sin(theta) : Trigonometry
  u cos(psi) : Product  SaturateOnIntegerOverflow=on  OutDataTypeStr=Inherit: Same as first input
  u sin(psi) : Product  SaturateOnIntegerOverflow=on  OutDataTypeStr=Inherit: Same as first input
  x : Outport
  y : Outport  Port=2
  psi : Outport  Port=3
  wires:
  yaw0/1 -> Sum2/2
  reset2/1 -> Discrete-Time Integrator1/2
  reset1/1 -> Discrete-Time Integrator/2
  reset/1 -> Discrete-Time Integrator2/2
  u sin(psi)/1 -> Sum1/1
  cos(psi)/1 -> u cos(psi)/1, a w cos(psi)/1
  w/1 -> a w cos(psi)/2, a w sin(psi)/2, Discrete-Time Integrator2/1
  Constant/1 -> a w sin(psi)/1, a w cos(psi)/3
  Discrete-Time Integrator/1 -> x/1
  Sum/1 -> Discrete-Time Integrator/1
  sin(theta)/1 -> a w sin(psi)/3, u sin(psi)/1
  a w cos(psi)/1 -> Sum1/2
  Sum2/1 -> psi/1, sin(theta)/1, cos(psi)/1
  u cos(psi)/1 -> Sum/2
  u/1 -> u sin(psi)/2, u cos(psi)/2
  a w sin(psi)/1 -> Sum/1
  Sum1/1 -> Discrete-Time Integrator1/1
  Discrete-Time Integrator1/1 -> y/1
  Discrete-Time Integrator2/1 -> Sum2/1

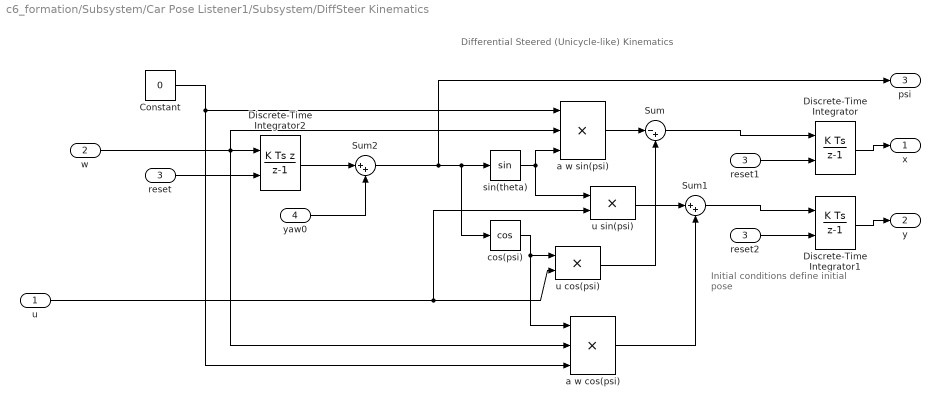
== system c6_formation/Subsystem/Car Pose Listener1/Subsystem/DiffSteer Kinematics ==
  note: Initial conditions define
      | initial pose
  note: Differential Steered (Unicycle-like) Kinematics
  u : Inport
  w : Inport  Port=2
  reset : Inport  Port=3
  yaw0 : Inport  Port=4
  Constant : Constant  Value=0
  Discrete-Time Integrator : DiscreteIntegrator  ExternalReset=falling  SampleTime=-1  ICPrevOutput=DiscIntNeverNeededParam  ICPrevScaledInput=DiscIntNeverNeededParam
  Discrete-Time Integrator1 : DiscreteIntegrator  ExternalReset=falling  SampleTime=-1  ICPrevOutput=DiscIntNeverNeededParam  ICPrevScaledInput=DiscIntNeverNeededParam
  Discrete-Time Integrator2 : DiscreteIntegrator  IntegratorMethod=Integration: Backward Euler  ExternalReset=falling  SampleTime=-1  ICPrevOutput=DiscIntNeverNeededParam  ICPrevScaledInput=DiscIntNeverNeededParam
  Sum : Sum  Inputs=|-+  SaturateOnIntegerOverflow=on
  Sum1 : Sum  Inputs=|++  SaturateOnIntegerOverflow=on
  Sum2 : Sum  Inputs=|++
  a w cos(psi) : Product  Inputs=3  SaturateOnIntegerOverflow=on  OutDataTypeStr=Inherit: Same as first input
  a w sin(psi) : Product  Inputs=3  SaturateOnIntegerOverflow=on  OutDataTypeStr=Inherit: Same as first input
  cos(psi) : Trigonometry  Operator=cos
  reset1 : InportShadow  Port=3
  reset2 : InportShadow  Port=3
  sin(theta) : Trigonometry
  u cos(psi) : Product  SaturateOnIntegerOverflow=on  OutDataTypeStr=Inherit: Same as first input
  u sin(psi) : Product  SaturateOnIntegerOverflow=on  OutDataTypeStr=Inherit: Same as first input
  x : Outport
  y : Outport  Port=2
  psi : Outport  Port=3
  wires:
  yaw0/1 -> Sum2/2
  reset2/1 -> Discrete-Time Integrator1/2
  reset1/1 -> Discrete-Time Integrator/2
  reset/1 -> Discrete-Time Integrator2/2
  u sin(psi)/1 -> Sum1/1
  cos(psi)/1 -> u cos(psi)/1, a w cos(psi)/1
  w/1 -> a w cos(psi)/2, a w sin(psi)/2, Discrete-Time Integrator2/1
  Constant/1 -> a w sin(psi)/1, a w cos(psi)/3
  Discrete-Time Integrator/1 -> x/1
  Sum/1 -> Discrete-Time Integrator/1
  sin(theta)/1 -> a w sin(psi)/3, u sin(psi)/1
  a w cos(psi)/1 -> Sum1/2
  Sum2/1 -> psi/1, sin(theta)/1, cos(psi)/1
  u cos(psi)/1 -> Sum/2
  u/1 -> u sin(psi)/2, u cos(psi)/2
  a w sin(psi)/1 -> Sum/1
  Sum1/1 -> Discrete-Time Integrator1/1
  Discrete-Time Integrator1/1 -> y/1
  Discrete-Time Integrator2/1 -> Sum2/1
